simulink model "Batman_Code"  (Simulink 7.8)
settings: Solver=FixedStepDiscrete  StartTime=0.0  StopTime=3  FixedStep=0.000250  RelTol=1e-3
InitFcn:
  | if (rtwenvironmentmode(bdroot(gcbh)) || ...
  |       exist('sldvisactive','file')~=0 && ...
  |       sldvisactive(bdroot(gcbh)) )
  |    ; %Simulation
  | else
  |   SendTargetStop(); %RTW-Build
  | end
undefined symbols (not defined in the file): A, A_T, B, BlockLoadFcnInfoBlock, CellNo, I_max_line, I_min_line, max_delta_V_cell, p, P_0, Q, R, R_i, T_max_cell, T_min_cell, V_max_bat, V_max_cell, V_min_bat, V_min_cell
libraries: c280xlib x19, lucasnuelle x2, idelinklib_ticcs x1, c2833xlib x1, idelinklib_tgtpref x1, idelinklib_common x1
(part 2 of 2)

== matlab function CAN-Receive/Function-Call Subsystem1/CAN_Daten_verwenden/Volt_02 ==
  data: msg input double; cell_voltages_in input double; cell_voltages_out output double
function cell_voltages_out = fcn(msg, cell_voltages_in)
% Datenempfang über CAN

% Auslesen der CAN-Nachricht
x1 = uint16(bitand(uint32(65535),bitshift(msg(1),-0)));
x2 = uint16(bitand(uint32(65535),bitshift(msg(1),-16)));
x3 = uint16(bitand(uint32(65535),bitshift(msg(2),-0)));
x4 = uint16(bitand(uint32(65535),bitshift(msg(2),-16)));


cell_voltages_in(5) = x1;
cell_voltages_in(6) = x2;
cell_voltages_in(7) = x3;
cell_voltages_in(8) = x4;

% Ausgabe
cell_voltages_out = cell_voltages_in;

== matlab function CAN-Transmit/(Daten verschicken) ==
  data: trig_0 output double; can_low_0 output double; can_high_0 output double; trig_1 output double; cell_voltages_in input double; cell_temperatures_in input double; SoC_in input double; can_low_1 output double; voltage_in input double; can_high_1 output double; trig_2 output double; current_in input double; can_low_2 output double; can_high_2 output double; trig_3 output double; can_low_3 output double; can_high_3 output double; trig_4 output double; can_low_4 output double; can_high_4 output double; trig_5 output double; can_low_5 output double; can_high_5 output double; trig_6 output double; can_low_6 output double; can_high_6 output double; trig_7 output double; can_low_7 output double; can_high_7 output double; trig_8 output double; can_low_8 output double; can_high_8 output double; error_code_out output double; error_index_out output double; balance_vec_in input double; bat_mode input double; error_code_in input double; error_index_in input double; error_in input double; lol1 input double; lol2 input double; error_out output double; CellNo parameter double
function [trig_0, can_low_0, can_high_0,trig_1, can_low_1, can_high_1, trig_2, can_low_2, can_high_2, trig_3, can_low_3, can_high_3, trig_4, can_low_4, can_high_4, trig_5, can_low_5, can_high_5, trig_6, can_low_6, can_high_6, trig_7, can_low_7, can_high_7, trig_8, can_low_8, can_high_8, error_code_out, error_index_out, error_out]= fcn(cell_voltages_in, cell_temperatures_in, SoC_in, voltage_in, current_in, balance_vec_in, bat_mode, error_code_in, error_index_in, error_in, lol1, lol2, CellNo)

persistent timer;
if isempty(timer)
    timer = uint8(1);
end
msg = uint32(0);

trig_0 = false;
trig_1 = false;
trig_2 = false;
trig_3 = false;
trig_4 = false;
trig_5 = false;
trig_6 = false;
trig_7 = false;
trig_8 = false;

can_low_0 = uint32(0);
can_high_0 = uint32(0);
can_low_1 = uint32(0);
can_high_1 = uint32(0);
can_low_2 = uint32(0);
can_high_2 = uint32(0);
can_low_3 = uint32(0);
can_high_3 = uint32(0);
can_low_4 = uint32(0);
can_high_4 = uint32(0);
can_low_5 = uint32(0);
can_high_5 = uint32(0);
can_low_6 = uint32(0);
can_high_6 = uint32(0);
can_low_7 = uint32(0);
can_high_7 = uint32(0);
can_low_8 = uint32(0);
can_high_8 = uint32(0);


if (error_in == 1)                                                         % Fehlernachricht verschicken   
    msg_1 = uint32(error_code_in);
    msg_2 = uint32(error_index_in);  
    msg_3 = uint32(0);
    msg_4 = uint32(error_in);
    msg_0_1 = uint32(bitor(msg_1,bitshift(msg_2,16)));
    msg_0_2 = uint32(bitor(msg_3,bitshift(msg_4,16)));
    can_low_0 = uint32(msg_0_1);
    can_high_0 = uint32(msg_0_2);
    trig_0 = true;  
    error_code_in = uint8(0);
    error_in = uint8(0);
    error_index_in = uint8(0);
elseif (error_in == 2)                                                         % Fehlernachricht verschicken
    msg_1 = uint32(0);
    msg_2 = uint32(0);
    msg_3 = uint32(0);
    msg_4 = uint32(0);
    msg_0_1 = uint32(bitor(msg_1,bitshift(msg_2,16)));
    msg_0_2 = uint32(bitor(msg_3,bitshift(msg_4,16)));
    can_low_0 = uint32(msg_0_1);
    can_high_0 = uint32(msg_0_2);
    trig_0 = true;
    error_code_in = uint8(0);
    error_in = uint8(0);
    error_index_in = uint8(0);
end

if (timer == 1)                                                            % Zellspannungen verschicken  
    msg_1 = uint32(cell_voltages_in(1));
    msg_2 = uint32(cell_voltages_in(2));  
    msg_3 = uint32(cell_voltages_in(3));
    msg_4 = uint32(cell_voltages_in(4));
    msg_1_1 = uint32(bitor(msg_1,bitshift(msg_2,16)));
    msg_1_2 = uint32(bitor(msg_3,bitshift(msg_4,16)));
    can_low_1 = uint32(msg_1_1);
    can_high_1 = uint32(msg_1_2);
    trig_1 = true;
end
    
if (timer == 2) 
    msg_5 = uint32(cell_voltages_in(5));
    msg_6 = uint32(cell_voltages_in(6));  
    msg_7 = uint32(cell_voltages_in(7));
    msg_8 = uint32(cell_voltages_in(8));
    msg_2_1 = uint32(bitor(msg_5,bitshift(msg_6,16)));
    msg_2_2 = uint32(bitor(msg_7,bitshift(msg_8,16)));
    can_low_2 = uint32(msg_2_1);
    can_high_2 = uint32(msg_2_2);
    trig_2 = true;
end

if (timer == 3)     
    msg_9 = uint32(cell_voltages_in(9));
    msg_10 = uint32(cell_voltages_in(10));  
    msg_11 = uint32(cell_voltages_in(11));
    msg_12 = uint32(cell_voltages_in(12));
    msg_3_1 = uint32(bitor(msg_9,bitshift(msg_10,16)));
    msg_3_2 = uint32(bitor(msg_11,bitshift(msg_12,16)));
    can_low_3 = uint32(msg_3_1);
    can_high_3 = uint32(msg_3_2);
    trig_3 = true;
end

if (timer == 4)                                                            % Zelltemperaturen verschicken  
    msg_1 = uint32(cell_temperatures_in(1));
    msg_2 = uint32(cell_temperatures_in(2));  
    msg_3 = uint32(cell_temperatures_in(3));
    msg_4 = uint32(cell_temperatures_in(4));
    msg_4_1 = uint32(bitor(msg_1,bitshift(msg_2,16)));
    msg_4_2 = uint32(bitor(msg_3,bitshift(msg_4,16)));
    can_low_4 = uint32(msg_4_1);
    can_high_4 = uint32(msg_4_2);
    trig_4 = true;
end

if (timer == 5) 
    msg_5 = uint32(cell_temperatures_in(5));
    msg_6 = uint32(cell_temperatures_in(6));  
    msg_7 = uint32(cell_temperatures_in(7));
    msg_8 = uint32(cell_temperatures_in(8));
    msg_5_1 = uint32(bitor(msg_5,bitshift(msg_6,16)));
    msg_5_2 = uint32(bitor(msg_7,bitshift(msg_8,16)));
    can_low_5 = uint32(msg_5_1);
    can_high_5 = uint32(msg_5_2);
    trig_5 = true;
end

if (timer == 6) 
    msg_9 = uint32(cell_temperatures_in(9));
    msg_10 = uint32(cell_temperatures_in(10));  
    msg_11 = uint32(cell_temperatures_in(11));
    msg_12 = uint32(cell_temperatures_in(12));
    msg_6_1 = uint32(bitor(msg_9,bitshift(msg_10,16)));
    msg_6_2 = uint32(bitor(msg_11,bitshift(msg_12,16)));
    can_low_6 = uint32(msg_6_1);
    can_high_6 = uint32(msg_6_2);
    trig_6 = true;
end

if (timer == 7)                                                            % SoC, Spannung, Strom verschicken 
    msg_1 = uint32(SoC_in);
    msg_2 = uint32(voltage_in);  
    msg_3 = uint32(current_in);
    msg_4 = uint32(bat_mode);
    msg_7_1 = uint32(bitor(msg_1,bitshift(msg_2,16)));
    msg_7_2 = uint32(bitor(msg_3,bitshift(msg_4,16)));   
    can_low_7 = uint32(msg_7_1);
    can_high_7 = uint32(msg_7_2);
    trig_7 = true;   
end

if (timer == 8)                                                            % Balance-Vector verschicken  
    for i = 1:1:CellNo
        if (balance_vec_in(i) == 1)
            msg = bitor(msg,bitshift(uint32(1),i-1));
        else
            msg = bitand(msg,bitcmp(bitshift(uint32(1),i-1)));
        end
    end
    msg_1 = uint32(msg);
    msg_2 = uint32(0);  
    msg_3 = uint32(lol1);
    msg_4 = uint32(lol2);
    msg_8_1 = uint32(bitor(msg_1,bitshift(msg_2,16)));
    msg_8_2 = uint32(bitor(msg_3,bitshift(msg_4,16)));   
    can_low_8 = uint32(msg_8_1);
    can_high_8 = uint32(msg_8_2);
    trig_8 = true;   
end

timer = timer + 1;                                                         % Timer hochzählen lassen

if (timer > 8)                                                             % Timer nach 8 Runden zurücksetzen
    timer = uint8(1);
end

% Ausgabe
error_code_out = error_code_in;
error_index_out = error_index_in;
error_out = error_in;

== matlab function CAN-Receive/Function-Call Subsystem3/data ==
  data: current_RTPC_out output double; voltage_RTPC_out output double; msg input double; bat_mode_out output double; operation_mode_out output double
function [current_RTPC_out, voltage_RTPC_out, bat_mode_out, operation_mode_out] = fcn(msg)
% Datenempfang über CAN

% Auslesen der CAN-Nachricht
x1 = int16(bitand(uint32(65535),bitshift(msg(1),-0)));  % operation_mode
x2 = int16(bitand(uint32(65535),bitshift(msg(1),-16))); % U_bat
x3 = int16(bitand(uint32(65535),bitshift(msg(2),-0)));  % I_bat
x4 = int16(bitand(uint32(65535),bitshift(msg(2),-16))); % bat_mode

operation_mode = uint16(x1);
voltage = uint16(x2);
current = int16(x3);
bat_mode = uint16(x4);


% Ausgabe
operation_mode_out = operation_mode;
voltage_RTPC_out = voltage;
current_RTPC_out = current;
bat_mode_out =  bat_mode;

== matlab function CAN-Receive/Function-Call Subsystem2/CAN_Daten_verwenden/Volt_03 ==
  data: msg input double; cell_voltages_in input double; cell_voltages_out output double
function cell_voltages_out = fcn(msg, cell_voltages_in)
% Datenempfang über CAN

% Auslesen der CAN-Nachricht
x1 = uint16(bitand(uint32(65535),bitshift(msg(1),-0)));
x2 = uint16(bitand(uint32(65535),bitshift(msg(1),-16)));
x3 = uint16(bitand(uint32(65535),bitshift(msg(2),-0)));
x4 = uint16(bitand(uint32(65535),bitshift(msg(2),-16)));

cell_voltages_in(9) = x1;
cell_voltages_in(10) = x2;
cell_voltages_in(11) = x3;
cell_voltages_in(12) = x4;

% Ausgabe
cell_voltages_out = cell_voltages_in;

== matlab function Limit Monitoring Balancing/balancing algorithm [mV] ==
  data: cell_voltage_in input uint16; balance_vec_out output uint8; CellNo parameter double; max_delta_V_cell parameter double
function balance_vec_out  = fcn(cell_voltage_in, CellNo, max_delta_V_cell)
% balancing algorithm

% initialization

persistent balance_vec;
if isempty(balance_vec)
    balance_vec=uint8(zeros(1,12));
end;
    
% Output
balance_vec_out = balance_vec;

== matlab function CAN-Receive/Function-Call Subsystem4/CAN_Daten_verwenden/Temp_01 ==
  data: msg input double; cell_temperatures_in input double; cell_temperatures_out output double
function cell_temperatures_out = fcn(msg, cell_temperatures_in)
% Datenempfang über CAN


% Auslesen der CAN-Nachricht
x1 = uint16(bitand(uint32(65535),bitshift(msg(1),-0)));
x2 = uint16(bitand(uint32(65535),bitshift(msg(1),-16)));
x3 = uint16(bitand(uint32(65535),bitshift(msg(2),-0)));
x4 = uint16(bitand(uint32(65535),bitshift(msg(2),-16)));

cell_temperatures_in(1) = x1;
cell_temperatures_in(2) = x2;
cell_temperatures_in(3) = x3;
cell_temperatures_in(4) = x4;


% Ausgabe
cell_temperatures_out = cell_temperatures_in;

== matlab function CAN-Receive/Function-Call Subsystem5/CAN_Daten_verwenden/Temp_02 ==
  data: msg input double; cell_temperatures_in input double; cell_temperatures_out output double
function cell_temperatures_out = fcn(msg, cell_temperatures_in)
% Datenempfang über CAN


% Auslesen der CAN-Nachricht
x1 = uint16(bitand(uint32(65535),bitshift(msg(1),-0)));
x2 = uint16(bitand(uint32(65535),bitshift(msg(1),-16)));
x3 = uint16(bitand(uint32(65535),bitshift(msg(2),-0)));
x4 = uint16(bitand(uint32(65535),bitshift(msg(2),-16)));

cell_temperatures_in(5) = x1;
cell_temperatures_in(6) = x2;
cell_temperatures_in(7) = x3;
cell_temperatures_in(8) = x4;


% Ausgabe
cell_temperatures_out = cell_temperatures_in;

== matlab function CAN-Receive/Function-Call Subsystem6/CAN_Daten_verwenden/Temp_03 ==
  data: msg input double; cell_temperatures_in input double; cell_temperatures_out output double
function cell_temperatures_out = fcn(msg, cell_temperatures_in)
% Datenempfang über CAN


% Auslesen der CAN-Nachricht
x1 = uint16(bitand(uint32(65535),bitshift(msg(1),-0)));
x2 = uint16(bitand(uint32(65535),bitshift(msg(1),-16)));
x3 = uint16(bitand(uint32(65535),bitshift(msg(2),-0)));
x4 = uint16(bitand(uint32(65535),bitshift(msg(2),-16)));

cell_temperatures_in(9) = x1;
cell_temperatures_in(10) = x2;
cell_temperatures_in(11) = x3;
cell_temperatures_in(12) = x4;


% Ausgabe
cell_temperatures_out = cell_temperatures_in;

== matlab function Limit Monitoring Balancing/limit monitoring [mV] / [K] / [mA] ==
  data: cell_voltage_in input uint16; cell_temperatures_in input double; current_in input double; voltage_in input double; CellNo parameter double; error_out output uint8; error_code_out output boolean; I_min_line parameter double; I_max_line parameter double; V_min_cell parameter double; V_max_cell parameter double; T_min_cell parameter double; T_max_cell parameter double; V_min_bat parameter double; V_max_bat parameter double; error_index_out output double
function [error_out, error_code_out, error_index_out] = fcn(cell_voltage_in, cell_temperatures_in, current_in, voltage_in, CellNo, I_min_line, I_max_line, V_min_cell, V_max_cell, T_min_cell, T_max_cell, V_min_bat, V_max_bat)

% initialization
persistent timer;
if isempty(timer)
    timer = uint8(1);
end

persistent error;
if isempty(error)
    error = uint8(0);
end

persistent error_code;
if isempty(error_code)
    error_code = uint8(0);
end

persistent error_index;
if isempty(error_index)
    error_index = uint8(0);
end

% Output
error_out = error;
error_code_out = error_code;
error_index_out = error_index;

== matlab function SoC_Estimation/Gesamtstrom Gesamtspannung1 ==
  data: bat_mode_in input double; current_out output double; current_in input double
function current_out = fcn(bat_mode_in, current_in)
% This block supports the Embedded MATLAB subset.
% See the help menu for details. 

if (bat_mode_in == 0)
    current_out = current_in;
else
    current_out = (current_in)*(-1);
end

== matlab function CAN-Receive/Function-Call Subsystem/CAN_Daten_verwenden/Volt_01 ==
  data: msg input double; cell_voltages_in input double; cell_voltages_out output double
function cell_voltages_out = fcn(msg, cell_voltages_in)
% Datenempfang über CAN

% Auslesen der CAN-Nachricht
x1 = uint16(bitand(uint32(65535),bitshift(msg(1),-0)));
x2 = uint16(bitand(uint32(65535),bitshift(msg(1),-16)));
x3 = uint16(bitand(uint32(65535),bitshift(msg(2),-0)));
x4 = uint16(bitand(uint32(65535),bitshift(msg(2),-16)));


cell_voltages_in(1) = x1;
cell_voltages_in(2) = x2;
cell_voltages_in(3) = x3;
cell_voltages_in(4) = x4;

% Ausgabe
cell_voltages_out = cell_voltages_in;

== matlab function SoC_Estimation/Extended Kalman Filter [mA] /  [mV]1 ==
  data: I_k input single; SoC output single; V_k input single; A parameter single; A_T parameter single; B parameter single; Q parameter single; R parameter single; R_i parameter single; p parameter single; P_0 parameter single
function SoC  = EKF(I_k, V_k, A, A_T, B, Q, R, R_i, p, P_0)

% 1) Initialization    
    persistent P;
   if isempty(P)
       P=0;
   end;
    persistent xk;
   if isempty(xk)
       xk=0;
   end;
    
% Output SoC
    if(100*xk(1)>100)
       SoC = single(100);
    elseif(100*xk(1)<0)
        SoC = single(0);
    else
        SoC = single(100*xk(1));   
    end;

== matlab function SoC_Estimation/battery_current [mA] battery_voltage [mV] ==
  data: current_out output double; currents_in input double; voltages_in input double; voltage_out output double
function [current_out, voltage_out]= fcn(currents_in, voltages_in)

% calculation battery voltage and battery current
voltage = uint16(sum(voltages_in)); % summation of cell voltages of a string
current = int16(mean(currents_in)); % summation of string currents


% Output
current_out = current;
voltage_out = voltage;
